simulink subsystem "Controls"  (R2024b)
settings: Solver=VariableStepAuto  StartTime=0.0  StopTime=10.0  RelTol=1e-3
undefined symbols (not defined in the file): D1, DiscIntNeverNeededParam, lag, Tctrl, test_alpha, Ts, Yg
libraries: powerlib_extras x74, simulink x10
(part 3 of 7)

== system Controls/Pole 2 Rectifier Control and Protection/Polarity_check ==
  converter_position : Inport
  Vdc_line : Inport  Port=2
  Vdc_neutral : Inport  Port=3
  Idc_in : Inport  Port=4
  Add : Sum  Inputs=+-
  Constant : Constant
  Constant1 : Constant  Value=-1
  Constant2 : Constant  Value=3
  Discrete 1st-Order Filter : powerlib_extras/Discrete  Control Blocks/Discrete 1st-Order Filter  FilterType=Lowpass  Tc=5  Ts=Tctrl  Initialize=off  Vac_Init=[0.8 -25 60]  Vdc_Init=-0.4  PlotResponse=off  param1=[1 500 0.1]
  MinMax : MinMax  Function=max  SampleTime=Tctrl
  Multiport Switch : MultiPortSwitch  DataPortOrder=Zero-based contiguous  Inputs=2  zeroidx=on  SaturateOnIntegerOverflow=off  InputSameDT=off
  Mux : Mux  Inputs=2
  Product : Product  RndMeth=Zero
  Product1 : Product  RndMeth=Zero
  Product2 : Product  RndMeth=Zero
  Relational Operator : RelationalOperator  OutDataTypeStr=boolean  InputSameDT=off
  Vdc_meas : Outport
  Idc_meas : Outport  Port=2
  wires:
  Product2/1 -> Idc_meas/1
  Relational Operator/1 -> Multiport Switch/1
  Constant2/1 -> Relational Operator/2
  converter_position/1 -> Relational Operator/1
  Idc_in/1 -> Product2/2
  Multiport Switch/1 -> Product2/1, Product1/1, Product/1
  Constant1/1 -> Multiport Switch/3
  Constant/1 -> Multiport Switch/2
  Vdc_neutral/1 -> Product1/2
  Product1/1 -> Discrete 1st-Order Filter/1
  Product/1 -> Mux/1, Add/1
  Vdc_line/1 -> Product/2
  MinMax/1 -> Vdc_meas/1
  Mux/1 -> MinMax/1
  Add/1 -> Mux/2
  Discrete 1st-Order Filter/1 -> Add/2

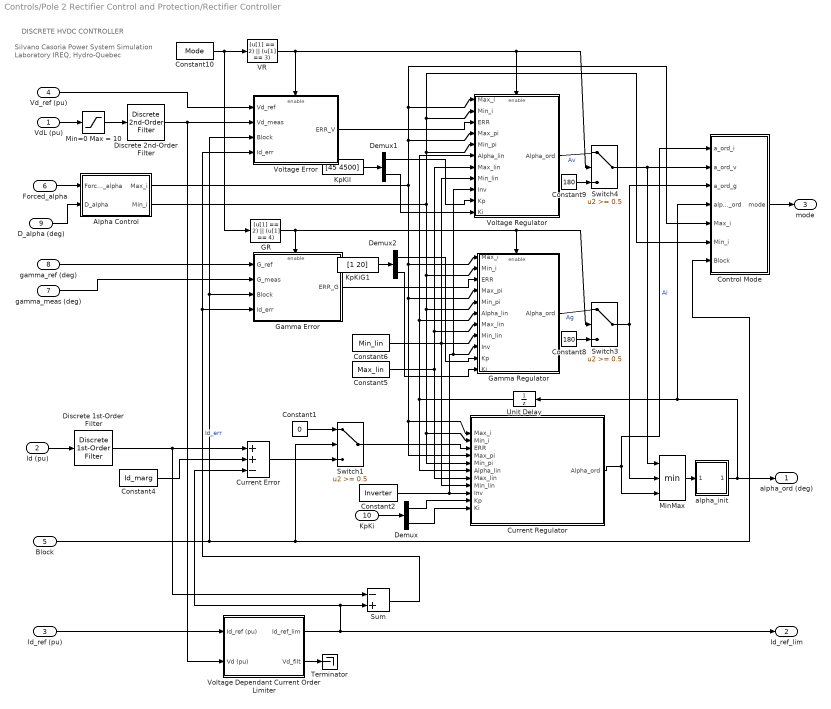
== system Controls/Pole 2 Rectifier Control and Protection/Rectifier Controller ==
  note: Silvano Casoria
      | Power System Simulation Laboratory
      |  IREQ, Hydro-Quebec
  note: DISCRETE HVDC CONTROLLER
  VdL (pu) : Inport
  Id (pu) : Inport  Port=2
  Id_ref (pu) : Inport  Port=3
  Vd_ref (pu) : Inport  Port=4
  Block : Inport  Port=5
  Forced_alpha : Inport  Port=6
  gamma_meas (deg) : Inport  Port=7
  gamma_ref (deg) : Inport  Port=8
  D_alpha (deg) : Inport  Port=9
  KpKi : Inport  Port=10
  Alpha Control : Subsystem
  Constant1 : Constant  Value=0
  Constant10 : Constant  Value=Mode
  Constant2 : Constant  Value=Inverter
  Constant4 : Constant  Value=Id_marg
  Constant5 : Constant  Value=Max_lin
  Constant6 : Constant  Value=Min_lin
  Constant8 : Constant  Value=180
  Constant9 : Constant  Value=180
  "Control Mode " : Subsystem
  Current Error : Sum  Inputs=++-  InputSameDT=on  SaturateOnIntegerOverflow=on  OutDataTypeStr=Inherit: Same as first input
  Current Regulator : Subsystem  mask(PI Regulator  With  External  Limits (Discrete)){Kp=Kp_I, Ki=Ki_I, IC_i=ICi_I, On_lin=on, dt=dt}
      mask prompts: Kp "Kp (deg/pu):"; Ki "Ki (deg/pu/s):"; IC_i "Integrator Initial Condition (deg):"; On_lin "Linearization  (On)"; dt "Sample time (s):"
      mask help: For the linearization it is important to specifie the mode of operation i.e. rectifier or inverter (negation of rectifier).
      mask Display: disp('PI Regulator\nWith external limits\n(Linearized Kp)\n(Discrete)\n\n')
  Demux : Demux  Outputs=2
  Demux1 : Demux  Outputs=2
  Demux2 : Demux  Outputs=2
  Discrete 1st-Order Filter : powerlib_extras/Discrete  Control Blocks/Discrete 1st-Order Filter  FilterType=Lowpass  Tc=T_I  Ts=dt  Initialize=off  Vac_Init=[0.8 -25 60]  Vdc_Init=-0.4  PlotResponse=off  param1=[1 500 0.1]
  Discrete 2nd-Order Filter : powerlib_extras/Discrete  Control Blocks/Discrete  2nd-Order Filter  FilterType=Lowpass  Fo=f0_V  Zeta=Z_V  Ts=dt  Initialize=off  Vac_Init=[0.8 -25 60]  Vdc_Init=-0.4  PlotResponse=off  param1=[1 500 1]
  GR : Fcn  Expr=(u[1] == 2) || (u[1] == 4)
  Gamma Error : Subsystem  TreatAsAtomicUnit=on
  Gamma Regulator : Subsystem  TreatAsAtomicUnit=on
  KpKiG1 : Constant  Value=[1 20]  OutDataTypeStr=double
  KpKiI : Constant  Value=[45 4500]
  Min=0 Max = 10 : Saturate  UpperLimit=10  LowerLimit=0
  MinMax : MinMax  Inputs=3  InputSameDT=on  SaturateOnIntegerOverflow=on
  Sum : Sum  Inputs=-+  InputSameDT=on  SaturateOnIntegerOverflow=on  OutDataTypeStr=Inherit: Same as first input
  Switch1 : Switch  Threshold=0.5
  Switch3 : Switch  Threshold=0.5
  Switch4 : Switch  Threshold=0.5
  Terminator : Terminator
  Unit Delay : UnitDelay  SampleTime=dt  HasFrameUpgradeWarning=on
  VR : Fcn  Expr=(u[1] == 2) || (u[1] == 3)
  Voltage Dependant Current Order Limiter : Subsystem  mask(Voltage Dependent Current Order Limiter  (Discrete)){Vd_seuil=Vd_seuil, Vd_min=Vd_min, Id_min=Id_min, Id_min_abs=Id_min_abs, Tu=Tup, pas=dt}
      mask prompts: Vd_seuil "Vd seuil (pu):"; Vd_min "Vd min (pu):"; Id_min "Id min (pu):"; Id_min_abs "Id min abs (pu):"; Tu "Up Time constant (s):"; pas "Sample time (s):"
      mask Display: disp('VDCOL\n (Discrete)')
  Voltage Error : Subsystem  TreatAsAtomicUnit=on
  Voltage Regulator : Subsystem  TreatAsAtomicUnit=on
  alpha_init : Subsystem
  alpha_ord (deg) : Outport
  Id_ref_lim : Outport  Port=2
  mode : Outport  Port=3
  wires:
  Demux/1 -> Current Regulator/10(Kp)
  Demux/2 -> Current Regulator/11(Ki)
  Demux2/1 -> Gamma Regulator/10(Kp)
  Demux2/2 -> Gamma Regulator/11(Ki)
  KpKiG1/1 -> Demux2/1
  Demux1/1 -> Voltage Regulator/10(Kp)
  Demux1/2 -> Voltage Regulator/11(Ki)
  KpKiI/1 -> Demux1/1
  KpKi/1 -> Demux/1
  Forced_alpha/1 -> Alpha Control/1(Forced_alpha)
  "Control Mode "/1(mode) -> mode/1
  Voltage Error/1(ERR_V) -> Voltage Regulator/3(ERR)
  Vd_ref (pu)/1 -> Voltage Error/1(Vd_ref)
  Sum/1 -> Gamma Error/4(Id_err), Voltage Error/4(Id_err)  "Id_err"
  gamma_meas (deg)/1 -> Gamma Error/2(G_meas)
  gamma_ref (deg)/1 -> Gamma Error/1(G_ref)
  Gamma Error/1(ERR_G) -> Gamma Regulator/3(ERR)
  Constant1/1 -> Switch1/1
  Switch4/1 -> "Control Mode "/2(a_ord_v), MinMax/1
  Switch3/1 -> "Control Mode "/3(a_ord_g), MinMax/2
  Current Regulator/1(Alpha_ord) -> "Control Mode "/1("a_ord_i "), MinMax/3  "Ai"
  Constant9/1 -> Switch4/3
  Voltage Regulator/1(Alpha_ord) -> Switch4/1  "Av"
  Constant8/1 -> Switch3/3
  Gamma Regulator/1(Alpha_ord) -> Switch3/1  "Ag"
  Switch1/1 -> Current Regulator/3(ERR)
  Constant2/1 -> Current Regulator/9(Inv), Gamma Regulator/9(Inv), Voltage Regulator/9(Inv)
  Block/1 -> Voltage Error/3(Block), Gamma Error/3(Block), "Control Mode "/7(Block), Switch1/2
  Alpha Control/2(Min_i) -> Voltage Regulator/5(Min_pi), "Control Mode "/6(Min_i), Voltage Regulator/2(Min_i), Gamma Regulator/2(Min_i), Gamma Regulator/5(Min_pi), Current Regulator/2(Min_i), Current Regulator/5(Min_pi)
  Constant5/1 -> Current Regulator/7(Max_lin), Voltage Regulator/7(Max_lin), Gamma Regulator/7(Max_lin)
  alpha_init/1(Out1) -> "Control Mode "/4(alpha_ord), Unit Delay/1, alpha_ord (deg)/1
  Unit Delay/1 -> Current Regulator/6(Alpha_lin), Voltage Regulator/6(Alpha_lin), Gamma Regulator/6(Alpha_lin)
  MinMax/1 -> alpha_init/1(In1)
  Current Error/1 -> Switch1/3
  Discrete 1st-Order Filter/1 -> Current Error/1, Sum/1
  Id (pu)/1 -> Discrete 1st-Order Filter/1
  VdL (pu)/1 -> Min=0 Max = 10/1
  Min=0 Max = 10/1 -> Discrete 2nd-Order Filter/1
  Discrete 2nd-Order Filter/1 -> Voltage Error/2(Vd_meas), Voltage Dependant Current Order Limiter/2(Vd (pu))
  Voltage Dependant Current Order Limiter/1(Id_ref_lim) -> Current Error/3, Sum/2, Id_ref_lim/1
  Voltage Dependant Current Order Limiter/2(Vd_filt) -> Terminator/1
  Id_ref (pu)/1 -> Voltage Dependant Current Order Limiter/1(Id_ref (pu))
  Constant4/1 -> Current Error/2
  Constant6/1 -> Current Regulator/8(Min_lin), Voltage Regulator/8(Min_lin), Gamma Regulator/8(Min_lin)
  Alpha Control/1(Max_i) -> Voltage Regulator/4(Max_pi), "Control Mode "/5(Max_i), Voltage Regulator/1(Max_i), Gamma Regulator/1(Max_i), Gamma Regulator/4(Max_pi), Current Regulator/1(Max_i), Current Regulator/4(Max_pi)
  D_alpha (deg)/1 -> Alpha Control/2(D_alpha)
  VR/1 -> Voltage Regulator/Enable, Switch4/2, Voltage Error/Enable
  Constant10/1 -> GR/1, VR/1
  GR/1 -> Gamma Regulator/Enable, Switch3/2, Gamma Error/Enable

== system Controls/Pole 2 Rectifier Control and Protection/Rectifier Protections ==
  note: DC Protections (in Rectifier)
  Uabc (pu) : Inport
  VdL (pu) : Inport  Port=2
  Deblocked : Inport  Port=3
  Low_ac_volt_oth : Inport  Port=4
  1st-Order T=3.3 ms : powerlib_extras/Discrete  Control Blocks/Discrete 1st-Order Filter  FilterType=Lowpass  Tc=0.0033  Ts=Tctrl  Initialize=off  Vac_Init=[0.8 -25 60]  Vdc_Init=-0.4  PlotResponse=off  param1=[1 500 0.1]
  DC Fault Protection (DCPROT) : Subsystem  mask(DC fault protection (in Rectifier)){STATE=on, Ref1=0.5, T1=0.070, T2=0.05, polarity=Positive, dt=Ts}
      mask prompts: STATE "ON State"; Ref1 "Detection level (pu):"; T1 "Detection delay (s):"; T2 "Forced alpha duration (s):"; polarity "Voltage polarity:"; dt "Sample time (s):"
      mask help:
      | The protection is active in the rectifier. It will detect a fault on the DC side and will force the delay angle into the inverter region in order to extinguish the fault current.
      |      The fault detection on the DC line is based on the drop in the line to ground voltage.
      |      The normal voltage polarity (+ or -) of the line is a parameter as well as the reference level (Detection level) of the fault detection.
      |      A delay time (Detection delay) is used in the detection to descriminate between a line fault and other disturbances resulting in a low DC voltage.
      |      A delay time (200 ms) is allowed, after the DC system start-up, before activating the detection logic to make sure that the normal operating DC voltage is established.
      |      Also, an external signal (Lock) generated by another protective function (e.g. Low AC voltage detection) will lock the detection for a minimum amount of time (set by an Off Delay bloc) in order to descriminate between any fault causing a low DC voltage.
      |      A detection will triger a Forced alpha during an ajustable interval (Forced alpha duration) sufficient to allow for deionization of the fault path prior to re-application of voltage.
      |
      |      In order to minimize the simulation time, an enabled susbystem having a sample time of  2 (ms) has been used in accordance with an acceptable precision.
      mask init:
      | if (polarity == 1)
      | 	sign = 1;
      | else
      | 	sign = -1;
      | end
      | 
      | if (STATE)
      | 	str = 'ON';
      | else
      | 	str = 'OFF';
      | end
      mask TypeOptions polarity: Positive | Negative
      mask Display: disp(['\n\n\n\nState:[',str,']'])
  Informations : Subsystem
      mask Display: disp('?')
  Logical Operator6 : Logic  Operator=OR
  Low AC Voltage Detection (LACVD) : Subsystem  TreatAsAtomicUnit=on  mask(Low AC voltage detection){STATE=on, Ref_1=0.70, dt=Ts}
      mask prompts: STATE "ON State"; Ref_1 "Detection level (pu):"; dt "Sample time (s):"
      mask help:
      | This bloc detects a low AC voltage condition on the commutation busbar and is used in the DC protection scheme. Its purpose is to descriminate between a drop in the AC voltage caused by a fault on the DC line or by a fault on the AC side.
      |
      |      An AC fault detection (Low_ac_voltage output signal) will occur when the AC voltage input (recified three-phase AC voltage) drops below a certain reference value (Detection level).
      |
      |      In order to minimize the simulation time, an enabled susbystem having a sample time of 1 (ms) has been used in accordance with an acceptable precision.
      mask init:
      | if (STATE)
      | 	str = 'ON';
      | else
      | 	str = 'OFF';
      | end
      mask Display: disp(['\n\n\n\nState:[',str,']'])
  Udio_6p : Subsystem
  Forced_alpha : Outport
  Low_ac_voltage : Outport  Port=2
  wires:
  Deblocked/1 -> DC Fault Protection (DCPROT)/2(Deblocked)
  VdL (pu)/1 -> DC Fault Protection (DCPROT)/1(VdL (pu))
  Logical Operator6/1 -> DC Fault Protection (DCPROT)/3(Lock)
  Low_ac_volt_oth/1 -> Logical Operator6/2
  DC Fault Protection (DCPROT)/1(Forced_alpha) -> Forced_alpha/1
  Low AC Voltage Detection (LACVD)/1(Low_AC_Voltage) -> Low_ac_voltage/1, Logical Operator6/1
  Uabc (pu)/1 -> Udio_6p/1(Uabc (pu))
  Udio_6p/1(Udio_6p) -> 1st-Order T=3.3 ms/1
  1st-Order T=3.3 ms/1 -> Low AC Voltage Detection (LACVD)/1(Uac (pu))

== system Controls/fault_trigger/faultgen ==
  Tacq : Inport
  Tst_set : Inport  Port=2
  Tdr_set : Inport  Port=3
  pert_set : Inport  Port=4
  pulse : Inport  Port=5
  Constant : Constant
  Product : Product  RndMeth=Zero
  Subsystem : Subsystem
  Tdr : Subsystem
  Tst : Subsystem
  faultgen : Subsystem
  sawtooth : Subsystem
  fault : Outport
  pertb : Outport  Port=2
  trig : Outport  Port=3
  wires:
  Tdr_set/1 -> Tdr/1(T_p)  "fault duration set (1 duration;2 variation; 3 period)"
  Tst_set/1 -> Tst/1(T_p)  "start time set (1 Tst;2 variation; 3 period)"
  Constant/1 -> Product/2
  Product/1 -> fault/1  "fault signal"
  sawtooth/2(trig) -> trig/1  "trig signal"
  pulse/1 -> sawtooth/2(pules)  "synchronous pulse if no pulse, must connect to positive"
  Subsystem/1(pertb) -> pertb/1  "perturbation signal"
  pert_set/1 -> Subsystem/1(pertset)  "perturbation set: 1,(0 none/1 square/2 triangle);2,amplitude"
  faultgen/1(fault) -> Product/1
  Tacq/1 -> sawtooth/1(Taqu), Subsystem/2(Tacq)  "acqusiition period"
  Tdr/1(t) -> faultgen/3(Tdur)
  Tst/1(t) -> faultgen/2(Tstat)
  sawtooth/1(sawtooth) -> faultgen/1(t), Subsystem/3(swth)

== system Controls/paraconv/Kp//Ki-Ki to Kp Ki1 ==
  i : Inport
  Mux3 : Mux  Inputs=2
  Product11 : Product  Inputs=1  RndMeth=Zero
  Selector12 : Selector  InputPortWidth=2  IndexOptions=Index vector (dialog)  Indices=2  OutputSizes=1
  o : Outport
  wires:
  i/1 -> Selector12/1, Product11/1
  Product11/1 -> Mux3/1
  Selector12/1 -> Mux3/2
  Mux3/1 -> o/1

== system Controls/paraconv/Kp//Ki-Ki to Kp Ki2 ==
  i : Inport
  Mux3 : Mux  Inputs=2
  Product11 : Product  Inputs=1  RndMeth=Zero
  Selector12 : Selector  InputPortWidth=2  IndexOptions=Index vector (dialog)  Indices=2  OutputSizes=1
  o : Outport
  wires:
  Mux3/1 -> o/1
  Selector12/1 -> Mux3/2
  Product11/1 -> Mux3/1
  i/1 -> Product11/1, Selector12/1

== system Controls/paraconv/Kp//Ki-Ki to Kp Ki3 ==
  i : Inport
  Mux3 : Mux  Inputs=2
  Product11 : Product  Inputs=1  RndMeth=Zero
  Selector12 : Selector  InputPortWidth=2  IndexOptions=Index vector (dialog)  Indices=2  OutputSizes=1
  o : Outport
  wires:
  i/1 -> Selector12/1, Product11/1
  Product11/1 -> Mux3/1
  Selector12/1 -> Mux3/2
  Mux3/1 -> o/1

== system Controls/Master Control/Start//Stop/S1 ==
  Start : Inport
  Data Type Conversion : DataTypeConversion  OutDataTypeStr=double  SaturateOnIntegerOverflow=off  RndMeth=Floor
  Start-Stop Ramp : RateLimiter  RisingSlewLimit=SS_ramp*3  FallingSlewLimit=-SS_ramp*3  SampleTimeMode=inherited
  Out1 : Outport  InitialOutput=0
  wires:
  Data Type Conversion/1 -> Start-Stop Ramp/1
  Start-Stop Ramp/1 -> Out1/1
  Start/1 -> Data Type Conversion/1

== system Controls/Pole 1 Inverter Control and Protection/12-pulse Firing Control/PLL ==
  Vabc(pu) : Inport
  Constant : Constant  Value=2*pi/3
  Discrete 3-phase PLL : powerlib_extras/Discrete  Control Blocks/Discrete 3-phase PLL  Fmin=0.75 * PLL_f0  Par_Init="[PLL_ph  PLL_f0]"  ParK="[PLL_Kp  PLL_Ki]"  Ts=dt  AGC=off
  Sum : Sum  Inputs=|+-  SaturateOnIntegerOverflow=on
  Sum1 : Sum  Inputs=|++  SaturateOnIntegerOverflow=on
  Terminator : Terminator
  Trigonometric Function : Trigonometry
  Trigonometric Function1 : Trigonometry
  Trigonometric Function2 : Trigonometry
  Va : Outport
  Vb : Outport  Port=2
  Vc : Outport  Port=3
  Freq : Outport  Port=4
  wires:
  Discrete 3-phase PLL/3 -> Terminator/1
  Trigonometric Function2/1 -> Vc/1
  Trigonometric Function1/1 -> Vb/1
  Trigonometric Function/1 -> Va/1
  Sum1/1 -> Trigonometric Function2/1
  Constant/1 -> Sum/2, Sum1/2
  Sum/1 -> Trigonometric Function1/1
  Discrete 3-phase PLL/2 -> Sum1/1, Sum/1, Trigonometric Function/1
  Vabc(pu)/1 -> Discrete 3-phase PLL/1
  Discrete 3-phase PLL/1 -> Freq/1

== system Controls/Pole 1 Inverter Control and Protection/Inverter Current //Voltage//Gamma Controller /Alpha Control ==
  Forced_alpha : Inport
  D_alpha : Inport  Port=2
  Constant1 : Constant  Value=alpha_min
  Constant2 : Constant  Value=alpha_max
  Constant3 : Constant  Value=test_alpha
  Data Type Conversion : DataTypeConversion  OutDataTypeStr=boolean
  Logical Operator : Logic  Operator=OR
  "Rate Limiter " : RateLimiter  RisingSlewLimit=PRate_fix  FallingSlewLimit=NRate_fix  SampleTimeMode=inherited
  "Rate Limiter   " : RateLimiter  RisingSlewLimit=PRate_fix  FallingSlewLimit=NRate_fix  SampleTimeMode=inherited
  Sum : Sum  Inputs=-+  InputSameDT=on  SaturateOnIntegerOverflow=on  OutDataTypeStr=Inherit: Same as first input
  Switch : Switch  Threshold=0.5
  Switch1 : Switch  Threshold=0.5
  fixed alpha (deg) : Constant  Value=alpha_fix
  Max_i : Outport
  Min_i : Outport  Port=2
  wires:
  Data Type Conversion/1 -> Logical Operator/2
  Forced_alpha/1 -> Data Type Conversion/1
  fixed alpha (deg)/1 -> Switch1/1, Switch/1
  Switch1/1 -> "Rate Limiter   "/1
  Switch/1 -> "Rate Limiter "/1
  Constant1/1 -> Switch1/3
  Logical Operator/1 -> Switch1/2, Switch/2
  Constant3/1 -> Logical Operator/1
  Constant2/1 -> Sum/2
  Sum/1 -> Switch/3
  D_alpha/1 -> Sum/1
  "Rate Limiter "/1 -> Max_i/1
  "Rate Limiter   "/1 -> Min_i/1

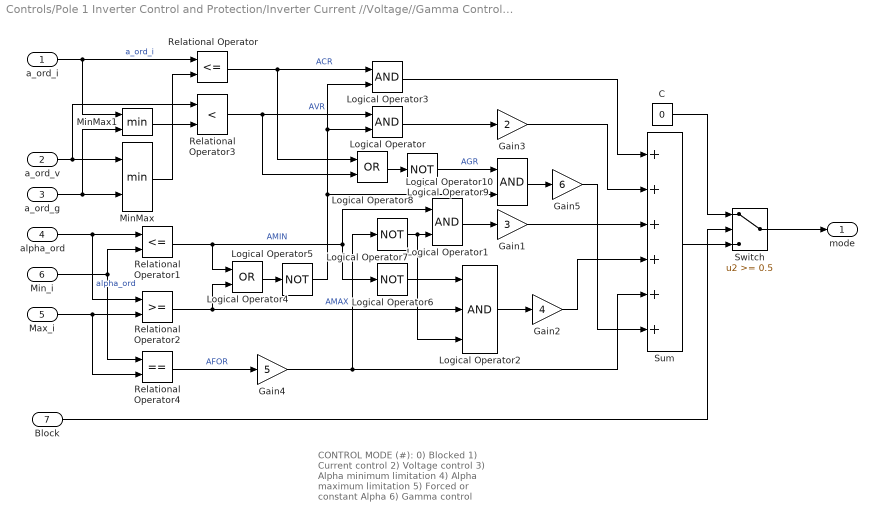
== system Controls/Pole 1 Inverter Control and Protection/Inverter Current //Voltage//Gamma Controller /Control Mode  ==
  note: CONTROL MODE (#):
      |
      | 0) Blocked
      | 1) Current control
      | 2) Voltage control
      | 3) Alpha minimum limitation
      | 4) Alpha maximum limitation
      | 5) Forced or constant Alpha
      | 6) Gamma control
  "a_ord_i " : Inport
  a_ord_v : Inport  Port=2
  a_ord_g : Inport  Port=3
  alpha_ord : Inport  Port=4
  Max_i : Inport  Port=5
  Min_i : Inport  Port=6
  Block : Inport  Port=7
  C : Constant  Value=0
  Gain1 : Gain  Gain=3  SaturateOnIntegerOverflow=on  OutDataTypeStr=Inherit: Same as input  ParamDataTypeStr=Inherit: Same as input
  Gain2 : Gain  Gain=4  SaturateOnIntegerOverflow=on  OutDataTypeStr=Inherit: Same as input  ParamDataTypeStr=Inherit: Same as input
  Gain3 : Gain  Gain=2  SaturateOnIntegerOverflow=on  OutDataTypeStr=Inherit: Same as input  ParamDataTypeStr=Inherit: Same as input
  Gain4 : Gain  Gain=5  SaturateOnIntegerOverflow=on  OutDataTypeStr=Inherit: Same as input  ParamDataTypeStr=Inherit: Same as input
  Gain5 : Gain  Gain=6  SaturateOnIntegerOverflow=on  OutDataTypeStr=Inherit: Same as input  ParamDataTypeStr=Inherit: Same as input
  Logical Operator{,1,3,10} (4 alike) : Logic
  Logical Operator2 : Logic  Inputs=3
  Logical Operator4 : Logic  Operator=OR
  Logical Operator{5..7,9} (4 alike) : Logic  Operator=NOT
  Logical Operator8 : Logic  Operator=OR
  MinMax : MinMax  Inputs=2  InputSameDT=on  SaturateOnIntegerOverflow=on
  MinMax1 : MinMax  Inputs=2  InputSameDT=on  SaturateOnIntegerOverflow=on
  Relational Operator : RelationalOperator  Operator=<=
  Relational Operator1 : RelationalOperator  Operator=<=
  Relational Operator2 : RelationalOperator
  Relational Operator3 : RelationalOperator  Operator=<
  Relational Operator4 : RelationalOperator  Operator===
  Sum : Sum  Inputs=++++++  InputSameDT=on  SaturateOnIntegerOverflow=on  OutDataTypeStr=Inherit: Same as first input
  Switch : Switch  Threshold=0.5
  mode : Outport
  wires:
  Logical Operator10/1 -> Gain5/1
  Logical Operator9/1 -> Logical Operator10/1  "AGR"
  MinMax1/1 -> Relational Operator3/2
  Gain5/1 -> Sum/6
  Logical Operator8/1 -> Logical Operator9/1
  MinMax/1 -> Relational Operator/2
  a_ord_g/1 -> MinMax1/2, MinMax/2
  a_ord_v/1 -> Relational Operator3/1, MinMax/1
  C/1 -> Switch/1
  Sum/1 -> Switch/3
  Switch/1 -> mode/1
  Block/1 -> Switch/2
  "a_ord_i "/1 -> MinMax1/1, Relational Operator/1  "a_ord_i"
  Relational Operator/1 -> Logical Operator8/1, Logical Operator3/1  "ACR"
  Logical Operator3/1 -> Sum/1
  Gain3/1 -> Sum/2
  Relational Operator3/1 -> Logical Operator8/2, Logical Operator/1  "AVR"
  Logical Operator/1 -> Gain3/1
  alpha_ord/1 -> Relational Operator1/1, Relational Operator2/1  "alpha_ord"
  Relational Operator1/1 -> Logical Operator4/1, Logical Operator6/1, Logical Operator1/1  "AMIN"
  Logical Operator4/1 -> Logical Operator5/1
  Relational Operator2/1 -> Logical Operator4/2, Logical Operator2/2  "AMAX"
  Logical Operator6/1 -> Logical Operator2/1
  Logical Operator2/1 -> Gain2/1
  Gain1/1 -> Sum/3
  Gain2/1 -> Sum/4
  Min_i/1 -> Relational Operator1/2, Relational Operator4/1
  Max_i/1 -> Relational Operator2/2, Relational Operator4/2
  Relational Operator4/1 -> Gain4/1  "AFOR"
  Logical Operator1/1 -> Gain1/1
  Gain4/1 -> Sum/5, Logical Operator7/1
  Logical Operator7/1 -> Logical Operator1/2, Logical Operator2/3
  Logical Operator5/1 -> Logical Operator10/2, Logical Operator/2, Logical Operator3/2

== system Controls/Pole 1 Inverter Control and Protection/Inverter Current //Voltage//Gamma Controller /Current Regulator ==
  note: PI Regulator With external limits (Linearized Kp) (Discrete)
  Max_i : Inport
  Min_i : Inport  Port=2
  ERR : Inport  Port=3
  Max_pi : Inport  Port=4
  Min_pi : Inport  Port=5
  Alpha_lin : Inport  Port=6
  Max_lin : Inport  Port=7
  Min_lin : Inport  Port=8
  Inv : Inport  Port=9
  Kp : Inport  Port=10
  Ki : Inport  Port=11
  Ground : Ground
  KI (deg per pu per s) : Gain  Gain=Ki  SaturateOnIntegerOverflow=on  OutDataTypeStr=Inherit: Same as input  ParamDataTypeStr=Inherit: Same as input
  Kp (deg per pu) : Constant  Value=Kp
  Kp Linearisation : Subsystem
  Prod : Product  InputSameDT=on  SaturateOnIntegerOverflow=on  OutDataTypeStr=Inherit: Same as first input
  Prod1 : Product  InputSameDT=on  SaturateOnIntegerOverflow=on  OutDataTypeStr=Inherit: Same as first input
  S16 : Subsystem  mask(Integrator  With  External  Dynamic  Limits (Discrete)){k=1, ic=IC_i, dt=dt}
      mask prompts: k "Gain:"; ic "Initial Condition:"; dt "Sample time: (s)"
      mask Display: disp('Integrator\nwith\nExternal Limits\nGain & Reset & Hold\n(Discrete)')
  S6 : Subsystem  mask(Limiter with External Limits){}
      mask Display: disp('      Limiter\n')
  Sum : Sum  InputSameDT=on  SaturateOnIntegerOverflow=on  OutDataTypeStr=Inherit: Same as first input
  Alpha_ord : Outport  InitialOutput=0
  wires:
  Prod1/1 -> S16/3(In)
  Ki/1 -> Prod1/2
  Kp/1 -> Kp Linearisation/2(Kp)
  Prod/1 -> Sum/1
  Min_lin/1 -> Kp Linearisation/4(Min_lin)
  Max_lin/1 -> Kp Linearisation/5(Max_lin)
  Inv/1 -> Kp Linearisation/3(Inv)
  Ground/1 -> S16/6(Reset Value), S16/5(Hold), S16/4(Reset)
  ERR/1 -> Prod1/1, Prod/2, KI (deg per pu per s)/1
  S16/1(Out) -> Sum/2
  Min_pi/1 -> S6/3(MIN)
  Max_pi/1 -> S6/1(MAX)
  Sum/1 -> S6/2(In)
  Min_i/1 -> S16/2(Min)
  Max_i/1 -> S16/1(Max)
  Kp Linearisation/1(Kp_lin) -> Prod/1
  S6/1("  ") -> Alpha_ord/1
  Alpha_lin/1 -> Kp Linearisation/1(Alpha_lin)

== system Controls/Pole 1 Inverter Control and Protection/Inverter Current //Voltage//Gamma Controller /Gamma Error ==
  G_ref : Inport
  G_meas : Inport  Port=2
  Block : Inport  Port=3
  Id_err : Inport  Port=4
  Enable : EnablePort
  Constant1 : Constant  Value=0
  Constant2 : Constant  Value=0
  Constant3 : Constant  Value=G_marg
  Constant4 : Constant  Value=Id_marg
  Discrete 1st-Order Filter : powerlib_extras/Discrete  Control Blocks/Discrete 1st-Order Filter  FilterType=Highpass  Tc=0.01  Ts=dt  Initialize=off  Vac_Init=[0.8 -25 60]  Vdc_Init=-0.4  PlotResponse=off  param1=[1 500 0.1]
  MIN:eps MAX:inf : Saturate  UpperLimit=inf  LowerLimit=eps
  Math Function : Math  Operator=reciprocal  SignedPower=on
  Product1 : Product  Inputs=3  InputSameDT=on  SaturateOnIntegerOverflow=on  OutDataTypeStr=Inherit: Same as first input
  S6 : Subsystem  mask(Limiter with External Limits){}
      mask Display: disp('      Limiter\n')
  Sum3 : Sum  Inputs=-+-  InputSameDT=on  SaturateOnIntegerOverflow=on  OutDataTypeStr=Inherit: Same as first input
  Switch2 : Switch  Threshold=0.5
  ERR_G : Outport
  wires:
  Constant3/1 -> Product1/1
  Id_err/1 -> S6/2(In)
  Discrete 1st-Order Filter/1 -> Sum3/3  "dG"
  Product1/1 -> Discrete 1st-Order Filter/1
  Constant4/1 -> S6/1(MAX), MIN:eps MAX:inf/1
  MIN:eps MAX:inf/1 -> Math Function/1
  Math Function/1 -> Product1/2
  S6/1("  ") -> Product1/3
  Constant2/1 -> S6/3(MIN)
  Switch2/1 -> ERR_G/1  "ERR"
  Block/1 -> Switch2/2
  Constant1/1 -> Switch2/1
  G_meas/1 -> Sum3/2
  G_ref/1 -> Sum3/1
  Sum3/1 -> Switch2/3

== system Controls/Pole 1 Inverter Control and Protection/Inverter Current //Voltage//Gamma Controller /Gamma Regulator ==
  Max_i : Inport
  Min_i : Inport  Port=2
  ERR : Inport  Port=3
  Max_pi : Inport  Port=4
  Min_pi : Inport  Port=5
  Alpha_lin : Inport  Port=6
  Max_lin : Inport  Port=7
  Min_lin : Inport  Port=8
  Inv : Inport  Port=9
  Kp : Inport  Port=10
  Ki : Inport  Port=11
  Enable : EnablePort
  Gamma Regulator : Subsystem  mask(PI Regulator  With  External  Limits (Discrete)){Kp=Kp_G, Ki=Ki_G, IC_i=ICi_G, On_lin=on, pas=dt}
      mask prompts: Kp "Kp (deg/pu):"; Ki "Ki (deg/pu/s):"; IC_i "Integrator Initial Condition (deg):"; On_lin "Linearization  (On)"; pas "Sample time (s):"
      mask help: For the linearization it is important to specifie the mode of operation i.e. rectifier or inverter (negation of rectifier).
      mask Display: disp('PI Regulator\nWith external limits\n(Linearized Kp)\n(Discrete)\n\n')
  Alpha_ord : Outport
  wires:
  Ki/1 -> Gamma Regulator/11(Ki)
  Kp/1 -> Gamma Regulator/10(Kp)
  Inv/1 -> Gamma Regulator/9(Inv)
  Min_lin/1 -> Gamma Regulator/8(Min_lin)
  Max_lin/1 -> Gamma Regulator/7(Max_lin)
  Alpha_lin/1 -> Gamma Regulator/6(Alpha_lin)
  Min_pi/1 -> Gamma Regulator/5(Min_pi)
  Max_pi/1 -> Gamma Regulator/4(Max_pi)
  ERR/1 -> Gamma Regulator/3(ERR)
  Min_i/1 -> Gamma Regulator/2(Min_i)
  Max_i/1 -> Gamma Regulator/1(Max_i)
  Gamma Regulator/1(Alpha_ord) -> Alpha_ord/1

== system Controls/Pole 1 Inverter Control and Protection/Inverter Current //Voltage//Gamma Controller /Voltage Dependant Current Order Limiter ==
  note: Voltage Dependant Current Order Limiter (VDCOL) (Discrete)
  Id_ref (pu) : Inport
  Vd (pu) : Inport  Port=2
  Constant : Constant  Value=Id_min
  Constant1 : Constant  Value=Vd_min
  Constant2 : Constant  Value=Vd_seuil
  Constant3 : Constant
  Constant4 : Constant
  Constant5 : Constant  Value=Tu
  Logical Operator : Logic  Operator=NOT
  Math Function : Math  Operator=reciprocal  SignedPower=on
  Max = 10 Min=Id_min_abs : Saturate  UpperLimit=10  LowerLimit=Id_min_abs
  MinMax2 : MinMax  Function=max  Inputs=2  InputSameDT=on  SaturateOnIntegerOverflow=on
  MinMax3 : MinMax  Inputs=2  InputSameDT=on  SaturateOnIntegerOverflow=on
  PB_R : Subsystem  mask(Low Pass Filter With Reset (discrete: Zoh method, Forward Euler)){ic=1, dt=pas}
      mask prompts: ic "Initial condition:"; dt "Sample time (s)"
      mask help:
      | The output will be reset to the input value (Time constant = 0)  during the input (2) is True. The Time constant (T) is defined by
      | input (3).
      mask Display:
      | plot(0,0,100,100,[90,80,70,60,50,40,29,20,10],[60,55,52,55,60,65,67,65,60],[89,80,71,60,50,40,30,20,10],[40,35,32,35,40,45,47,45,40],[56,44],[70,50]);
      | disp('\n\nD')
  Product : Product  InputSameDT=on  SaturateOnIntegerOverflow=on
  Product1 : Product  InputSameDT=on  SaturateOnIntegerOverflow=on
  Product2 : Product  InputSameDT=on  SaturateOnIntegerOverflow=on  OutDataTypeStr=Inherit: Same as first input
  Product3 : Product  InputSameDT=on  SaturateOnIntegerOverflow=on  OutDataTypeStr=Inherit: Same as first input
  Product4 : Product  InputSameDT=on  SaturateOnIntegerOverflow=on  OutDataTypeStr=Inherit: Same as first input
  Relational Operator : RelationalOperator
  Sum : Sum  Inputs=+-  InputSameDT=on  SaturateOnIntegerOverflow=on  OutDataTypeStr=Inherit: Same as first input
  Sum1 : Sum  Inputs=+-  InputSameDT=on  SaturateOnIntegerOverflow=on  OutDataTypeStr=Inherit: Same as first input
  Sum2 : Sum  Inputs=+-  InputSameDT=on  SaturateOnIntegerOverflow=on  OutDataTypeStr=Inherit: Same as first input
  Sum3 : Sum  InputSameDT=on  SaturateOnIntegerOverflow=on  OutDataTypeStr=Inherit: Same as first input
  Unit Delay : UnitDelay  SampleTime=pas  HasFrameUpgradeWarning=on
  Id_ref_lim : Outport  InitialOutput=0
  Vd_filt : Outport  Port=2  InitialOutput=0
  wires:
  Logical Operator/1 -> PB_R/2(Reset)
  Unit Delay/1 -> Logical Operator/1
  Vd (pu)/1 -> Relational Operator/1, PB_R/1("In ")
  PB_R/1(Out) -> Relational Operator/2, Vd_filt/1, Product2/2
  Constant5/1 -> PB_R/3(T)
  Constant3/1 -> Sum/1
  Constant1/1 -> Sum1/2
  Sum1/1 -> Math Function/1
  Sum/1 -> Product/1
  Math Function/1 -> Product/2
  Constant4/1 -> Sum2/1
  Sum2/1 -> Sum3/1  "B"
  Product2/1 -> Sum3/2
  Sum3/1 -> Product1/2
  Constant/1 -> Sum/2, Product4/1
  Product4/1 -> Max = 10 Min=Id_min_abs/1  "min"
  Id_ref (pu)/1 -> Product1/1, MinMax3/1, Product4/2
  MinMax3/1 -> Id_ref_lim/1
  Product3/1 -> Sum2/2
  Product/1 -> Product2/1, Product3/2  "A"
  Constant2/1 -> Sum1/1, Product3/1
  Product1/1 -> MinMax2/1  "Idref_lim"
  MinMax2/1 -> MinMax3/2
  Max = 10 Min=Id_min_abs/1 -> MinMax2/2
  Relational Operator/1 -> Unit Delay/1

== system Controls/Pole 1 Inverter Control and Protection/Inverter Current //Voltage//Gamma Controller /Voltage Error ==
  Vd_ref : Inport
  Vd_meas : Inport  Port=2
  Block : Inport  Port=3
  Id_err : Inport  Port=4
  Enable : EnablePort
  Constant1 : Constant  Value=0
  Constant2 : Constant  Value=0
  Constant3 : Constant  Value=Vd_marg
  Constant4 : Constant  Value=Id_marg
  Discrete 1st-Order Filter : powerlib_extras/Discrete  Control Blocks/Discrete 1st-Order Filter  FilterType=Highpass  Tc=0.01  Ts=dt  Initialize=off  Vac_Init=[0.8 -25 60]  Vdc_Init=-0.4  PlotResponse=off  param1=[1 500 0.1]
  MIN:eps MAX:inf : Saturate  UpperLimit=inf  LowerLimit=eps
  Math Function : Math  Operator=reciprocal  SignedPower=on
  Product1 : Product  Inputs=3  InputSameDT=on  SaturateOnIntegerOverflow=on  OutDataTypeStr=Inherit: Same as first input
  S6 : Subsystem  mask(Limiter with External Limits){}
      mask Display: disp('      Limiter\n')
  Sum3 : Sum  Inputs=+--  InputSameDT=on  SaturateOnIntegerOverflow=on  OutDataTypeStr=Inherit: Same as first input
  Switch2 : Switch  Threshold=0.5
  ERR_V : Outport
  wires:
  Sum3/1 -> Switch2/3
  Vd_ref/1 -> Sum3/1
  Vd_meas/1 -> Sum3/2
  Constant1/1 -> Switch2/1
  Block/1 -> Switch2/2
  Switch2/1 -> ERR_V/1  "ERR"
  Constant2/1 -> S6/3(MIN)
  S6/1("  ") -> Product1/3
  Math Function/1 -> Product1/2
  MIN:eps MAX:inf/1 -> Math Function/1
  Constant4/1 -> MIN:eps MAX:inf/1, S6/1(MAX)
  Product1/1 -> Discrete 1st-Order Filter/1
  Discrete 1st-Order Filter/1 -> Sum3/3  "dV"
  Id_err/1 -> S6/2(In)
  Constant3/1 -> Product1/1

== system Controls/Pole 1 Inverter Control and Protection/Inverter Current //Voltage//Gamma Controller /Voltage Regulator ==
  Max_i : Inport
  Min_i : Inport  Port=2
  ERR : Inport  Port=3
  Max_pi : Inport  Port=4
  Min_pi : Inport  Port=5
  Alpha_lin : Inport  Port=6
  Max_lin : Inport  Port=7
  Min_lin : Inport  Port=8
  Inv : Inport  Port=9
  Kp : Inport  Port=10
  Ki : Inport  Port=11
  Enable : EnablePort
  Voltage Regulator : Subsystem  mask(PI Regulator  With  External  Limits (Discrete)){Kp=Kp_V, Ki=Ki_V, IC_i=ICi_V, On_lin=on, pas=dt}
      mask prompts: Kp "Kp (deg/pu):"; Ki "Ki (deg/pu/s):"; IC_i "Integrator Initial Condition (deg):"; On_lin "Linearization  (On)"; pas "Sample time (s):"
      mask help: For the linearization it is important to specifie the mode of operation i.e. rectifier or inverter (negation of rectifier).
      mask Display: disp('PI Regulator\nWith external limits\n(Linearized Kp)\n(Discrete)\n\n')
  Alpha_ord : Outport
  wires:
  Ki/1 -> Voltage Regulator/11(Ki)
  Kp/1 -> Voltage Regulator/10(Kp)
  Voltage Regulator/1(Alpha_ord) -> Alpha_ord/1
  Max_i/1 -> Voltage Regulator/1(Max_i)
  Min_i/1 -> Voltage Regulator/2(Min_i)
  ERR/1 -> Voltage Regulator/3(ERR)
  Max_pi/1 -> Voltage Regulator/4(Max_pi)
  Min_pi/1 -> Voltage Regulator/5(Min_pi)
  Alpha_lin/1 -> Voltage Regulator/6(Alpha_lin)
  Max_lin/1 -> Voltage Regulator/7(Max_lin)
  Min_lin/1 -> Voltage Regulator/8(Min_lin)
  Inv/1 -> Voltage Regulator/9(Inv)

== system Controls/Pole 1 Inverter Control and Protection/Inverter Current //Voltage//Gamma Controller /alpha_init ==
  In1 : Inport  PortDimensions=1
  IC : InitialCondition  Value=min([ICi_V,ICi_I,ICi_G])
  Out1 : Outport
  wires:
  In1/1 -> IC/1
  IC/1 -> Out1/1

== system Controls/Pole 1 Inverter Control and Protection/Inverter Protections/Commutation Failure Prevention Control (CFPREV) ==
  note: Commutation failure Prevention Control Module (CFPREV)
  Uabc (pu) : Inport
  C : Constant  Value=STATE
  Enabled Subsystem : Subsystem  TreatAsAtomicUnit=on
  AMIN_CFPREV (deg) : Outport
  wires:
  Enabled Subsystem/1(AMIN_CFPREV (deg)) -> AMIN_CFPREV (deg)/1
  Uabc (pu)/1 -> Enabled Subsystem/1(Uabc (pu))
  C/1 -> Enabled Subsystem/Enable

== system Controls/Pole 1 Inverter Control and Protection/Inverter Protections/Informations ==
  note: NOTE 1: Result of a failure of the incoming valve to take over the direct current before the commutating voltage reverses its polarity.
  note: DC Protections - Inverter
  note: DESCRIPTION
  note: The LACVD detects a low AC voltage condition on the inverter commutation bus and sends a signal
      | (Lock) to the DCPROT (in the rectifier) in order to prevent the detection of a DC fault when the drop in
      | the DC voltage is due to a fault on the AC side. The LACVD at the irectifier sends also a signal to
      | lock the DCPROT for the same reason.
  note: The Commutation failure prevention control (CFPREV) and the Low AC voltage detection (LACVD)
      | constitutes the protective functions at the rinverter.
  note: The CFPREV  mitigates commutation failures due to AC voltage dips. After a fault detection (three-phase or
      | one-phase) an angle value (AMIN_CFPREV) is sent to the converter control in order to be deducted from the
      | maximum delay angle limit (alpha_max). In practice, the commutation margin is consequently enlarged
      | reducing therefore the risk of commutation failures (note 1).

== system Controls/Pole 1 Inverter Control and Protection/Inverter Protections/Low AC Voltage Detection (LACVD) ==
  note: Low AC Voltage Detection
  Uac (pu) : Inport
  Enabled Subsystem : Subsystem  TreatAsAtomicUnit=on
  Low_AC_Voltage : Outport
  wires:
  Enabled Subsystem/1(Low_AC_Voltage) -> Low_AC_Voltage/1
  Uac (pu)/1 -> Enabled Subsystem/1(Uac (pu))

== system Controls/Pole 1 Inverter Control and Protection/Inverter Protections/Udio_6p ==
  note: Three-phase full-wave rectification
  note: Silvano Casoria
      | Power System Laboratory, IREQ
      | Hydro-Quebec
  Uabc (pu) : Inport
  MinMax : MinMax  Function=max  InputSameDT=on  SaturateOnIntegerOverflow=on
  MinMax1 : MinMax  InputSameDT=on  SaturateOnIntegerOverflow=on
  Sum : Sum  Inputs=+-  InputSameDT=on  SaturateOnIntegerOverflow=on  OutDataTypeStr=Inherit: Same as first input
  conversion pu ac->dc : Gain  Gain=pi/(3*sqrt(3))  SaturateOnIntegerOverflow=on  OutDataTypeStr=Inherit: Same as input  ParamDataTypeStr=Inherit: Same as input
  Udio_6p : Outport
  wires:
  conversion pu ac->dc/1 -> Udio_6p/1
  Sum/1 -> conversion pu ac->dc/1
  Uabc (pu)/1 -> MinMax1/1, MinMax/1
  MinMax/1 -> Sum/1
  MinMax1/1 -> Sum/2

== system Controls/Pole 1 Rectifier Control and Protection/12-pulse Firing Control/PLL ==
  Vabc(pu) : Inport
  Constant : Constant  Value=2*pi/3
  Discrete 3-phase PLL : powerlib_extras/Discrete  Control Blocks/Discrete 3-phase PLL  Fmin=0.75 * PLL_f0  Par_Init="[PLL_ph  PLL_f0]"  ParK="[PLL_Kp  PLL_Ki]"  Ts=dt  AGC=off
  Sum : Sum  Inputs=|+-  SaturateOnIntegerOverflow=on
  Sum1 : Sum  Inputs=|++  SaturateOnIntegerOverflow=on
  Terminator : Terminator
  Trigonometric Function : Trigonometry
  Trigonometric Function1 : Trigonometry
  Trigonometric Function2 : Trigonometry
  Va : Outport
  Vb : Outport  Port=2
  Vc : Outport  Port=3
  Freq : Outport  Port=4
  wires:
  Discrete 3-phase PLL/3 -> Terminator/1
  Trigonometric Function2/1 -> Vc/1
  Trigonometric Function1/1 -> Vb/1
  Trigonometric Function/1 -> Va/1
  Sum1/1 -> Trigonometric Function2/1
  Constant/1 -> Sum/2, Sum1/2
  Sum/1 -> Trigonometric Function1/1
  Discrete 3-phase PLL/2 -> Sum1/1, Sum/1, Trigonometric Function/1
  Vabc(pu)/1 -> Discrete 3-phase PLL/1
  Discrete 3-phase PLL/1 -> Freq/1

== system Controls/Pole 1 Rectifier Control and Protection/Rectifier Controller/Alpha Control ==
  Forced_alpha : Inport
  D_alpha : Inport  Port=2
  Constant1 : Constant  Value=alpha_min
  Constant2 : Constant  Value=alpha_max
  Constant3 : Constant  Value=test_alpha
  Data Type Conversion : DataTypeConversion  OutDataTypeStr=boolean
  Logical Operator : Logic  Operator=OR
  "Rate Limiter " : RateLimiter  RisingSlewLimit=PRate_fix  FallingSlewLimit=NRate_fix  SampleTimeMode=inherited
  "Rate Limiter   " : RateLimiter  RisingSlewLimit=PRate_fix  FallingSlewLimit=NRate_fix  SampleTimeMode=inherited
  Sum : Sum  Inputs=-+  InputSameDT=on  SaturateOnIntegerOverflow=on  OutDataTypeStr=Inherit: Same as first input
  Switch : Switch  Threshold=0.5
  Switch1 : Switch  Threshold=0.5
  fixed alpha (deg) : Constant  Value=alpha_fix
  Max_i : Outport
  Min_i : Outport  Port=2
  wires:
  Data Type Conversion/1 -> Logical Operator/2
  Forced_alpha/1 -> Data Type Conversion/1
  fixed alpha (deg)/1 -> Switch1/1, Switch/1
  Switch1/1 -> "Rate Limiter   "/1
  Switch/1 -> "Rate Limiter "/1
  Constant1/1 -> Switch1/3
  Logical Operator/1 -> Switch1/2, Switch/2
  Constant3/1 -> Logical Operator/1
  Constant2/1 -> Sum/2
  Sum/1 -> Switch/3
  D_alpha/1 -> Sum/1
  "Rate Limiter "/1 -> Max_i/1
  "Rate Limiter   "/1 -> Min_i/1

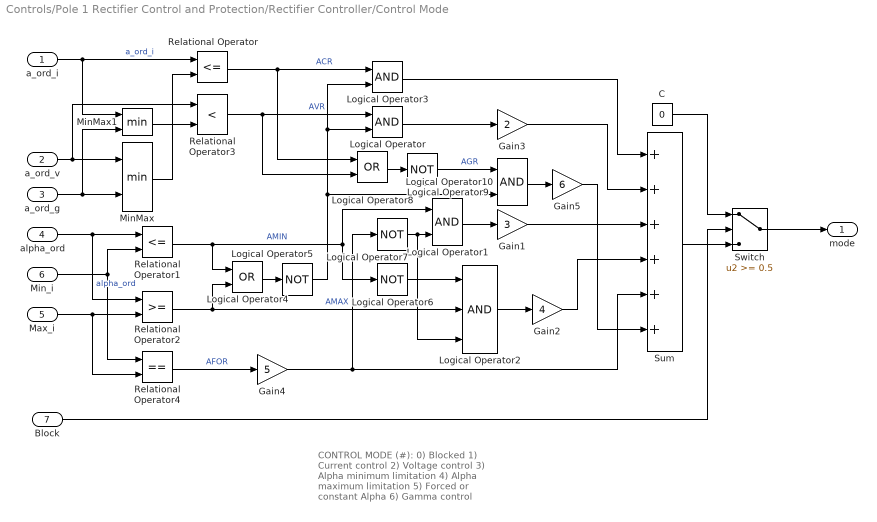
== system Controls/Pole 1 Rectifier Control and Protection/Rectifier Controller/Control Mode  ==
  note: CONTROL MODE (#):
      |
      | 0) Blocked
      | 1) Current control
      | 2) Voltage control
      | 3) Alpha minimum limitation
      | 4) Alpha maximum limitation
      | 5) Forced or constant Alpha
      | 6) Gamma control
  "a_ord_i " : Inport
  a_ord_v : Inport  Port=2
  a_ord_g : Inport  Port=3
  alpha_ord : Inport  Port=4
  Max_i : Inport  Port=5
  Min_i : Inport  Port=6
  Block : Inport  Port=7
  C : Constant  Value=0
  Gain1 : Gain  Gain=3  SaturateOnIntegerOverflow=on  OutDataTypeStr=Inherit: Same as input  ParamDataTypeStr=Inherit: Same as input
  Gain2 : Gain  Gain=4  SaturateOnIntegerOverflow=on  OutDataTypeStr=Inherit: Same as input  ParamDataTypeStr=Inherit: Same as input
  Gain3 : Gain  Gain=2  SaturateOnIntegerOverflow=on  OutDataTypeStr=Inherit: Same as input  ParamDataTypeStr=Inherit: Same as input
  Gain4 : Gain  Gain=5  SaturateOnIntegerOverflow=on  OutDataTypeStr=Inherit: Same as input  ParamDataTypeStr=Inherit: Same as input
  Gain5 : Gain  Gain=6  SaturateOnIntegerOverflow=on  OutDataTypeStr=Inherit: Same as input  ParamDataTypeStr=Inherit: Same as input
  Logical Operator{,1,3,10} (4 alike) : Logic
  Logical Operator2 : Logic  Inputs=3
  Logical Operator4 : Logic  Operator=OR
  Logical Operator{5..7,9} (4 alike) : Logic  Operator=NOT
  Logical Operator8 : Logic  Operator=OR
  MinMax : MinMax  Inputs=2  InputSameDT=on  SaturateOnIntegerOverflow=on
  MinMax1 : MinMax  Inputs=2  InputSameDT=on  SaturateOnIntegerOverflow=on
  Relational Operator : RelationalOperator  Operator=<=
  Relational Operator1 : RelationalOperator  Operator=<=
  Relational Operator2 : RelationalOperator
  Relational Operator3 : RelationalOperator  Operator=<
  Relational Operator4 : RelationalOperator  Operator===
  Sum : Sum  Inputs=++++++  InputSameDT=on  SaturateOnIntegerOverflow=on  OutDataTypeStr=Inherit: Same as first input
  Switch : Switch  Threshold=0.5
  mode : Outport
  wires:
  Logical Operator10/1 -> Gain5/1
  Logical Operator9/1 -> Logical Operator10/1  "AGR"
  MinMax1/1 -> Relational Operator3/2
  Gain5/1 -> Sum/6
  Logical Operator8/1 -> Logical Operator9/1
  MinMax/1 -> Relational Operator/2
  a_ord_g/1 -> MinMax1/2, MinMax/2
  a_ord_v/1 -> Relational Operator3/1, MinMax/1
  C/1 -> Switch/1
  Sum/1 -> Switch/3
  Switch/1 -> mode/1
  Block/1 -> Switch/2
  "a_ord_i "/1 -> MinMax1/1, Relational Operator/1  "a_ord_i"
  Relational Operator/1 -> Logical Operator8/1, Logical Operator3/1  "ACR"
  Logical Operator3/1 -> Sum/1
  Gain3/1 -> Sum/2
  Relational Operator3/1 -> Logical Operator8/2, Logical Operator/1  "AVR"
  Logical Operator/1 -> Gain3/1
  alpha_ord/1 -> Relational Operator1/1, Relational Operator2/1  "alpha_ord"
  Relational Operator1/1 -> Logical Operator4/1, Logical Operator6/1, Logical Operator1/1  "AMIN"
  Logical Operator4/1 -> Logical Operator5/1
  Relational Operator2/1 -> Logical Operator4/2, Logical Operator2/2  "AMAX"
  Logical Operator6/1 -> Logical Operator2/1
  Logical Operator2/1 -> Gain2/1
  Gain1/1 -> Sum/3
  Gain2/1 -> Sum/4
  Min_i/1 -> Relational Operator1/2, Relational Operator4/1
  Max_i/1 -> Relational Operator2/2, Relational Operator4/2
  Relational Operator4/1 -> Gain4/1  "AFOR"
  Logical Operator1/1 -> Gain1/1
  Gain4/1 -> Sum/5, Logical Operator7/1
  Logical Operator7/1 -> Logical Operator1/2, Logical Operator2/3
  Logical Operator5/1 -> Logical Operator10/2, Logical Operator/2, Logical Operator3/2

== system Controls/Pole 1 Rectifier Control and Protection/Rectifier Controller/Current Regulator ==
  note: PI Regulator With external limits (Linearized Kp) (Discrete)
  Max_i : Inport
  Min_i : Inport  Port=2
  ERR : Inport  Port=3
  Max_pi : Inport  Port=4
  Min_pi : Inport  Port=5
  Alpha_lin : Inport  Port=6
  Max_lin : Inport  Port=7
  Min_lin : Inport  Port=8
  Inv : Inport  Port=9
  Kp : Inport  Port=10
  Ki : Inport  Port=11
  Ground : Ground
  KI (deg per pu per s) : Gain  Gain=Ki  SaturateOnIntegerOverflow=on  OutDataTypeStr=Inherit: Same as input  ParamDataTypeStr=Inherit: Same as input
  Kp (deg per pu) : Constant  Value=Kp
  Kp Linearisation : Subsystem
  Prod : Product  InputSameDT=on  SaturateOnIntegerOverflow=on  OutDataTypeStr=Inherit: Same as first input
  Prod1 : Product  InputSameDT=on  SaturateOnIntegerOverflow=on  OutDataTypeStr=Inherit: Same as first input
  S16 : Subsystem  mask(Integrator  With  External  Dynamic  Limits (Discrete)){k=1, ic=IC_i, dt=dt}
      mask prompts: k "Gain:"; ic "Initial Condition:"; dt "Sample time: (s)"
      mask Display: disp('Integrator\nwith\nExternal Limits\nGain & Reset & Hold\n(Discrete)')
  S6 : Subsystem  mask(Limiter with External Limits){}
      mask Display: disp('      Limiter\n')
  Sum : Sum  InputSameDT=on  SaturateOnIntegerOverflow=on  OutDataTypeStr=Inherit: Same as first input
  Alpha_ord : Outport  InitialOutput=0
  wires:
  Prod1/1 -> S16/3(In)
  Ki/1 -> Prod1/2
  Kp/1 -> Kp Linearisation/2(Kp)
  Prod/1 -> Sum/1
  Min_lin/1 -> Kp Linearisation/4(Min_lin)
  Max_lin/1 -> Kp Linearisation/5(Max_lin)
  Inv/1 -> Kp Linearisation/3(Inv)
  Ground/1 -> S16/6(Reset Value), S16/5(Hold), S16/4(Reset)
  ERR/1 -> Prod1/1, Prod/2, KI (deg per pu per s)/1
  S16/1(Out) -> Sum/2
  Min_pi/1 -> S6/3(MIN)
  Max_pi/1 -> S6/1(MAX)
  Sum/1 -> S6/2(In)
  Min_i/1 -> S16/2(Min)
  Max_i/1 -> S16/1(Max)
  Kp Linearisation/1(Kp_lin) -> Prod/1
  S6/1("  ") -> Alpha_ord/1
  Alpha_lin/1 -> Kp Linearisation/1(Alpha_lin)

== system Controls/Pole 1 Rectifier Control and Protection/Rectifier Controller/Gamma Error ==
  G_ref : Inport
  G_meas : Inport  Port=2
  Block : Inport  Port=3
  Id_err : Inport  Port=4
  Enable : EnablePort
  Constant1 : Constant  Value=0
  Constant2 : Constant  Value=0
  Constant3 : Constant  Value=G_marg
  Constant4 : Constant  Value=Id_marg
  Discrete 1st-Order Filter : powerlib_extras/Discrete  Control Blocks/Discrete 1st-Order Filter  FilterType=Highpass  Tc=0.01  Ts=dt  Initialize=off  Vac_Init=[0.8 -25 60]  Vdc_Init=-0.4  PlotResponse=off  param1=[1 500 0.1]
  MIN:eps MAX:inf : Saturate  UpperLimit=inf  LowerLimit=eps
  Math Function : Math  Operator=reciprocal  SignedPower=on
  Product1 : Product  Inputs=3  InputSameDT=on  SaturateOnIntegerOverflow=on  OutDataTypeStr=Inherit: Same as first input
  S6 : Subsystem  mask(Limiter with External Limits){}
      mask Display: disp('      Limiter\n')
  Sum3 : Sum  Inputs=-+-  InputSameDT=on  SaturateOnIntegerOverflow=on  OutDataTypeStr=Inherit: Same as first input
  Switch2 : Switch  Threshold=0.5
  ERR_G : Outport
  wires:
  Constant3/1 -> Product1/1
  Id_err/1 -> S6/2(In)
  Discrete 1st-Order Filter/1 -> Sum3/3  "dG"
  Product1/1 -> Discrete 1st-Order Filter/1
  Constant4/1 -> S6/1(MAX), MIN:eps MAX:inf/1
  MIN:eps MAX:inf/1 -> Math Function/1
  Math Function/1 -> Product1/2
  S6/1("  ") -> Product1/3
  Constant2/1 -> S6/3(MIN)
  Switch2/1 -> ERR_G/1  "ERR"
  Block/1 -> Switch2/2
  Constant1/1 -> Switch2/1
  G_meas/1 -> Sum3/2
  G_ref/1 -> Sum3/1
  Sum3/1 -> Switch2/3

== system Controls/Pole 1 Rectifier Control and Protection/Rectifier Controller/Gamma Regulator ==
  Max_i : Inport
  Min_i : Inport  Port=2
  ERR : Inport  Port=3
  Max_pi : Inport  Port=4
  Min_pi : Inport  Port=5
  Alpha_lin : Inport  Port=6
  Max_lin : Inport  Port=7
  Min_lin : Inport  Port=8
  Inv : Inport  Port=9
  Kp : Inport  Port=10
  Ki : Inport  Port=11
  Enable : EnablePort
  Gamma Regulator : Subsystem  mask(PI Regulator  With  External  Limits (Discrete)){Kp=Kp_G, Ki=Ki_G, IC_i=ICi_G, On_lin=on, pas=dt}
      mask prompts: Kp "Kp (deg/pu):"; Ki "Ki (deg/pu/s):"; IC_i "Integrator Initial Condition (deg):"; On_lin "Linearization  (On)"; pas "Sample time (s):"
      mask help: For the linearization it is important to specifie the mode of operation i.e. rectifier or inverter (negation of rectifier).
      mask Display: disp('PI Regulator\nWith external limits\n(Linearized Kp)\n(Discrete)\n\n')
  Alpha_ord : Outport
  wires:
  Ki/1 -> Gamma Regulator/11(Ki)
  Kp/1 -> Gamma Regulator/10(Kp)
  Inv/1 -> Gamma Regulator/9(Inv)
  Min_lin/1 -> Gamma Regulator/8(Min_lin)
  Max_lin/1 -> Gamma Regulator/7(Max_lin)
  Alpha_lin/1 -> Gamma Regulator/6(Alpha_lin)
  Min_pi/1 -> Gamma Regulator/5(Min_pi)
  Max_pi/1 -> Gamma Regulator/4(Max_pi)
  ERR/1 -> Gamma Regulator/3(ERR)
  Min_i/1 -> Gamma Regulator/2(Min_i)
  Max_i/1 -> Gamma Regulator/1(Max_i)
  Gamma Regulator/1(Alpha_ord) -> Alpha_ord/1

== system Controls/Pole 1 Rectifier Control and Protection/Rectifier Controller/Voltage Dependant Current Order Limiter ==
  note: Voltage Dependant Current Order Limiter (VDCOL) (Discrete)
  Id_ref (pu) : Inport
  Vd (pu) : Inport  Port=2
  Constant : Constant  Value=Id_min
  Constant1 : Constant  Value=Vd_min
  Constant2 : Constant  Value=Vd_seuil
  Constant3 : Constant
  Constant4 : Constant
  Constant5 : Constant  Value=Tu
  Logical Operator : Logic  Operator=NOT
  Math Function : Math  Operator=reciprocal  SignedPower=on
  Max = 10 Min=Id_min_abs : Saturate  UpperLimit=10  LowerLimit=Id_min_abs
  MinMax2 : MinMax  Function=max  Inputs=2  InputSameDT=on  SaturateOnIntegerOverflow=on
  MinMax3 : MinMax  Inputs=2  InputSameDT=on  SaturateOnIntegerOverflow=on
  PB_R : Subsystem  mask(Low Pass Filter With Reset (discrete: Zoh method, Forward Euler)){ic=1, dt=pas}
      mask prompts: ic "Initial condition:"; dt "Sample time (s)"
      mask help:
      | The output will be reset to the input value (Time constant = 0)  during the input (2) is True. The Time constant (T) is defined by
      | input (3).
      mask Display:
      | plot(0,0,100,100,[90,80,70,60,50,40,29,20,10],[60,55,52,55,60,65,67,65,60],[89,80,71,60,50,40,30,20,10],[40,35,32,35,40,45,47,45,40],[56,44],[70,50]);
      | disp('\n\nD')
  Product : Product  InputSameDT=on  SaturateOnIntegerOverflow=on
  Product1 : Product  InputSameDT=on  SaturateOnIntegerOverflow=on
  Product2 : Product  InputSameDT=on  SaturateOnIntegerOverflow=on  OutDataTypeStr=Inherit: Same as first input
  Product3 : Product  InputSameDT=on  SaturateOnIntegerOverflow=on  OutDataTypeStr=Inherit: Same as first input
  Product4 : Product  InputSameDT=on  SaturateOnIntegerOverflow=on  OutDataTypeStr=Inherit: Same as first input
  Relational Operator : RelationalOperator
  Sum : Sum  Inputs=+-  InputSameDT=on  SaturateOnIntegerOverflow=on  OutDataTypeStr=Inherit: Same as first input
  Sum1 : Sum  Inputs=+-  InputSameDT=on  SaturateOnIntegerOverflow=on  OutDataTypeStr=Inherit: Same as first input
  Sum2 : Sum  Inputs=+-  InputSameDT=on  SaturateOnIntegerOverflow=on  OutDataTypeStr=Inherit: Same as first input
  Sum3 : Sum  InputSameDT=on  SaturateOnIntegerOverflow=on  OutDataTypeStr=Inherit: Same as first input
  Unit Delay : UnitDelay  SampleTime=pas  HasFrameUpgradeWarning=on
  Id_ref_lim : Outport  InitialOutput=0
  Vd_filt : Outport  Port=2  InitialOutput=0
  wires:
  Logical Operator/1 -> PB_R/2(Reset)
  Unit Delay/1 -> Logical Operator/1
  Vd (pu)/1 -> Relational Operator/1, PB_R/1("In ")
  PB_R/1(Out) -> Relational Operator/2, Vd_filt/1, Product2/2
  Constant5/1 -> PB_R/3(T)
  Constant3/1 -> Sum/1
  Constant1/1 -> Sum1/2
  Sum1/1 -> Math Function/1
  Sum/1 -> Product/1
  Math Function/1 -> Product/2
  Constant4/1 -> Sum2/1
  Sum2/1 -> Sum3/1  "B"
  Product2/1 -> Sum3/2
  Sum3/1 -> Product1/2
  Constant/1 -> Sum/2, Product4/1
  Product4/1 -> Max = 10 Min=Id_min_abs/1  "min"
  Id_ref (pu)/1 -> Product1/1, MinMax3/1, Product4/2
  MinMax3/1 -> Id_ref_lim/1
  Product3/1 -> Sum2/2
  Product/1 -> Product2/1, Product3/2  "A"
  Constant2/1 -> Sum1/1, Product3/1
  Product1/1 -> MinMax2/1  "Idref_lim"
  MinMax2/1 -> MinMax3/2
  Max = 10 Min=Id_min_abs/1 -> MinMax2/2
  Relational Operator/1 -> Unit Delay/1
